simulink model "Engine_Start_harness"  (Simulink 7.7)
settings: Solver=FixedStepDiscrete  SolverMode=SingleTasking  StartTime=0.0  StopTime=100  FixedStep=0.01  RelTol=1e-3
PostLoadFcn:
  | load EngineStart.mat
undefined symbols (not defined in the file): ACTIVE, INACTIVE, NORMAL, SA_ATTACHMENT, SA_SERVICE_TOOL, sigbuilder_block, srate
CloseFcn:
  | rtwprivate ssgencode ModelCloseRequest sle_main_controller
settings Model: Creator=smindema  LastModifiedBy=aliebel  RecordCoverage=on  CovMetricSettings=dcmw  CovCumulativeReport=on  CovModelRefEnable=off
settings MATStruct: SampleTime=0.01  Offset=0  Priority=[1.0]
settings DataIOCC: LimitDataPoints=off  SaveOutput=off  SaveTime=off
settings OptimizationCC: BlockReduction=off  InlineParams=on  ExpressionFolding=off  StateBitsets=on  DataBitsets=on  UseTempVars=on  InitFltsAndDblsToZero=on  NoFixptDivByZeroProtection=on  EfficientFloat2IntCast=on  OptimizeModelRefInitCode=on
settings DebuggingCC: SaveWithParameterizedLinksMsg=none  MultiTaskDSMMsg=warning  MultiTaskCondExecSysMsg=none  IntegerOverflowMsg=none  ModelReferenceCSMismatchMessage=warning
settings HardwareCC: ProdBitPerInt=16  ProdBitPerPointer=16  ProdIntDivRoundTo=Floor  ProdEndianess=BigEndian  ProdWordSize=16  ProdHWDeviceType=Motorola HC12
settings ModelReferenceCC: ModelReferenceNumInstancesAllowed=Single
settings RTWCC: SystemTargetFile=ert.tlc  GenCodeOnly=on  TemplateMakefile=ert_default_tmf  Description=Real-Time Workshop Embedded Coder (no auto configuration)  GenerateReport=on  RetainRTWFile=on  ProcessScript=ert_make_rtw_hook  IncludeHyperlinkInReport=on  LaunchReport=on  IncludeERTFirstTime=on
settings RTWCC: CustomHeaderCode=|
  | #include "cpp_req_defines.h"
  | #include "hw_fin.h"
  | #include "cdata.h"
settings CodeAppCC: IgnoreCustomStorageClasses=off  DefineNamingRule=UpperCase
settings ERTTargetCC: TargetFcnLib=ansi_tfl_tmw.mat  FunctionExecutionProfile=off  MultiwordLength=2048  GenerateSampleERTMain=on  IncludeMdlTerminateFcn=off  SupportAbsoluteTime=off  SupportNonFinite=off  SupportComplex=off  PurelyIntegerCode=on  ERTCustomFileTemplate=gen_rtw_req_defines_h.tlc  GlobalDataDefinition=InSeparateSourceFile  GlobalDataReference=InSeparateHeaderFile  ConvertIfToSwitch=off

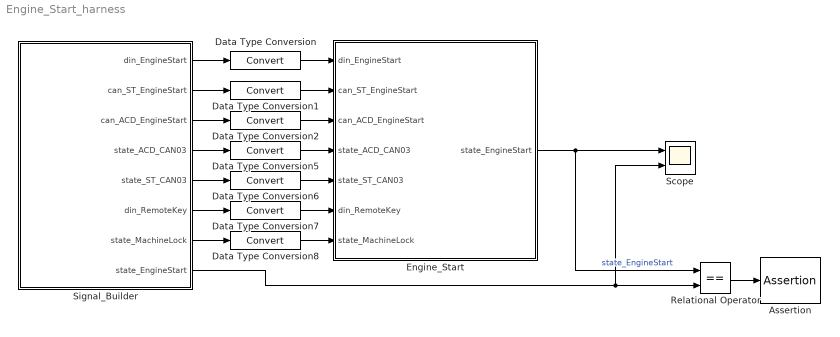
== system Engine_Start_harness ==
  Assertion : Assertion  Enabled=off
  Data Type Conversion{,1..2,5..8} (7 alike) : DataTypeConversion
  Engine_Start : Subsystem  TreatAsAtomicUnit=on  SystemSampleTime=srate  RTWFcnName=Engine_Start  RTWFileName=mod_Inputs
      settings: RTWSystemCode=Function  RTWFcnNameOpts=User specified  RTWFileNameOpts=User specified
  Relational Operator : RelationalOperator  Operator===  OutDataTypeStr=boolean
  Scope : Scope  NumInputPorts=2
      settings: YMin=-5~-5  YMax=5~5  MaxDataPoints=50000
  Signal_Builder : Subsystem  Tag=STV Subsys  LoadFcn=sigbuilder_block('load');  StartFcn=sigbuilder_block('start');  StopFcn=sigbuilder_block('stop');  ClipboardFcn=sigbuilder_block('clipboard');  mask(Sigbuilder block){}
      mask help: Sigbuilder GUI
      mask init:
      | if ~strcmp(get_param(bdroot(gcbh),'SimulationStatus'),'stopped') tuvar = sigbuilder_block('maskInit'); end
      settings: CopyFcn=sigbuilder_block('copy');  DeleteFcn=sigbuilder_block('delete');  ModelCloseFcn=sigbuilder_block('modelClose');  PreSaveFcn=sigbuilder_block('preSave');  NameChangeFcn=sigbuilder_block('namechange');  OpenFcn=sigbuilder_block('open',[91.5 225.75 1119.75 509.25 ]);  CloseFcn=sigbuilder_block('close');
      mask Display: plot(0,0,100,100,[10,10,40,40,10],[80,20,20,80,80],[40,10],[50,50], [40,27,10],[65,72,56],[40,25,25,10],[28,28,43,43]);
  wires:
  Engine_Start/1(state_EngineStart) -> Scope/1, Relational Operator/1  "state_EngineStart"
  Signal_Builder/1(din_EngineStart) -> Data Type Conversion/1
  Signal_Builder/2(can_ST_EngineStart) -> Data Type Conversion1/1
  Data Type Conversion/1 -> Engine_Start/1(din_EngineStart)
  Data Type Conversion1/1 -> Engine_Start/2(can_ST_EngineStart)
  Relational Operator/1 -> Assertion/1
  Data Type Conversion2/1 -> Engine_Start/3(can_ACD_EngineStart)
  Signal_Builder/3(can_ACD_EngineStart) -> Data Type Conversion2/1
  Signal_Builder/4(state_ACD_CAN03) -> Data Type Conversion5/1
  Signal_Builder/5(state_ST_CAN03) -> Data Type Conversion6/1
  Data Type Conversion5/1 -> Engine_Start/4(state_ACD_CAN03)
  Data Type Conversion6/1 -> Engine_Start/5(state_ST_CAN03)
  Signal_Builder/6(din_RemoteKey) -> Data Type Conversion7/1
  Signal_Builder/7(state_MachineLock) -> Data Type Conversion8/1
  Data Type Conversion7/1 -> Engine_Start/6(din_RemoteKey)
  Data Type Conversion8/1 -> Engine_Start/7(state_MachineLock)
  Signal_Builder/8(state_EngineStart) -> Relational Operator/2, Scope/2

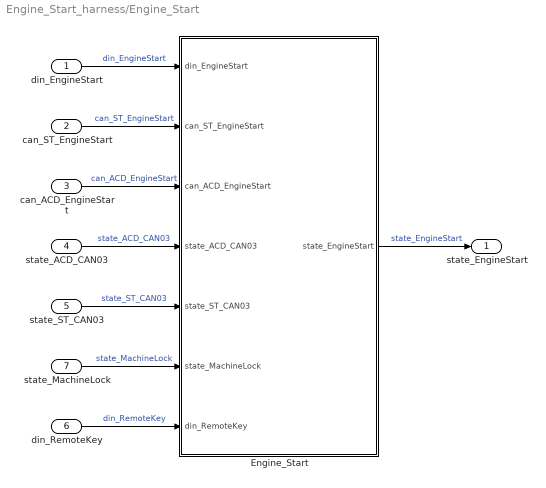
== system Engine_Start_harness/Engine_Start ==
  din_EngineStart : Inport
  can_ST_EngineStart : Inport  Port=2
  can_ACD_EngineStart : Inport  Port=3
  state_ACD_CAN03 : Inport  Port=4
  state_ST_CAN03 : Inport  Port=5
  din_RemoteKey : Inport  Port=6
  state_MachineLock : Inport  Port=7
  Engine_Start : Stateflow chart  TreatAsAtomicUnit=on
  state_EngineStart : Outport
  wires:
  Engine_Start/1(state_EngineStart) -> state_EngineStart/1  "state_EngineStart"
  din_EngineStart/1 -> Engine_Start/1(din_EngineStart)  "din_EngineStart"
  can_ST_EngineStart/1 -> Engine_Start/2(can_ST_EngineStart)  "can_ST_EngineStart"
  can_ACD_EngineStart/1 -> Engine_Start/3(can_ACD_EngineStart)  "can_ACD_EngineStart"
  state_ACD_CAN03/1 -> Engine_Start/4(state_ACD_CAN03)  "state_ACD_CAN03"
  state_ST_CAN03/1 -> Engine_Start/5(state_ST_CAN03)  "state_ST_CAN03"
  state_MachineLock/1 -> Engine_Start/6(state_MachineLock)  "state_MachineLock"
  din_RemoteKey/1 -> Engine_Start/7(din_RemoteKey)  "din_RemoteKey"

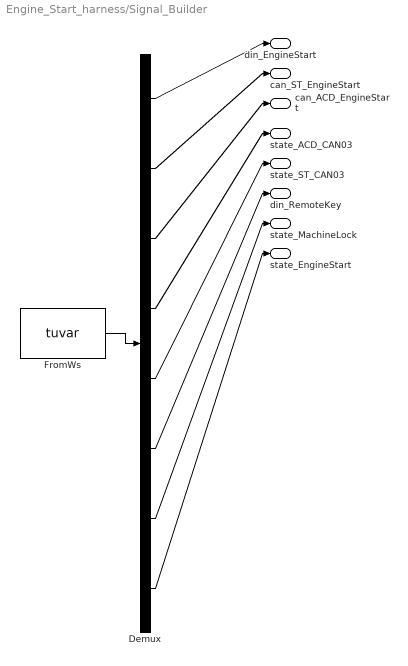
== system Engine_Start_harness/Signal_Builder ==
  Demux : Demux  Tag=STV Demux  Outputs=8
  FromWs : FromWorkspace  Tag=STV FromWs  VariableName=tuvar  SampleTime=0  SigBuilderData=DataTag0  VnvData=DataTag1
      SigBuilderData=|
      | common.afterFinalStr = 'Extrapolate'
      | common.sampleTime = 0
      | dataSet.timeRange = [0 100]
      | dataSet.name = 'T1-Key'
      | sbobj.Groups.Name = 'T1-Key'
      | sbobj.Groups.Signals(1).Name = 'din_EngineStart'
      | sbobj.Groups.Signals(1).XData = [0 4.8 4.8 8.3 8.3 13.9 13.9 17.8 17.8 23.7 23.7 28 28 100]
      | sbobj.Groups.Signals(1).YData = [0 0 1 1 0 0 1 1 0 0 1 1 0 0]
      | sbobj.Groups.Signals(2).Name = 'can_ST_EngineStart'
      | sbobj.Groups.Signals(2).XData = [0 30 30 35 35 40 40 45 45 100]
      | sbobj.Groups.Signals(2).YData = [0 0 1 1 0 0 1 1 0 0]
      | sbobj.Groups.Signals(3).Name = 'can_ACD_EngineStart'
      | sbobj.Groups.Signals(3).XData = [0 50 50 54.5 54.5 60 60 65 65 100]
      | sbobj.Groups.Signals(3).YData = [0 0 1 1 0 0 1 1 0 0]
      | sbobj.Groups.Signals(4).Name = 'state_ACD_CAN03'
      | sbobj.Groups.Signals(4).XData = [0 52 52 62.7 62.7 100]
      | sbobj.Groups.Signals(4).YData = [4 4 8 8 4 4]
      | sbobj.Groups.Signals(5).Name = 'state_ST_CAN03'
      | sbobj.Groups.Signals(5).XData = [0 32.8 32.8 42 42 100]
      | sbobj.Groups.Signals(5).YData = [4 4 8 8 4 4]
      | sbobj.Groups.Signals(6).Name = 'din_RemoteKey'
      | sbobj.Groups.Signals(6).XData = [0 11.1 11.1 19.8 19.8 100]
      | sbobj.Groups.Signals(6).YData = [0 0 1 1 0 0]
      | sbobj.Groups.Signals(7).Name = 'state_MachineLock'
      | sbobj.Groups.Signals(7).XData = [0 10 10 100]
      | sbobj.Groups.Signals(7).YData = [1 1 0 0]
      | sbobj.Groups.Signals(8).Name = 'state_EngineStart'
      | sbobj.Groups.Signals(8).XData = [0 23.71 23.71 28 28 32.81 32.81 35 35 40 40 42 42 52 52 54.5 54.5 60 60 62.7 62.7 100]
      | sbobj.Groups.Signals(8).YData = [0 0 1 1 0 0 1 1 0 0 1 1 0 0 1 1 0 0 1 1 0 0]
  din_EngineStart : Outport  Tag=STV Outport
  can_ST_EngineStart : Outport  Tag=STV Outport  Port=2
  can_ACD_EngineStart : Outport  Tag=STV Outport  Port=3
  state_ACD_CAN03 : Outport  Tag=STV Outport  Port=4
  state_ST_CAN03 : Outport  Tag=STV Outport  Port=5
  din_RemoteKey : Outport  Tag=STV Outport  Port=6
  state_MachineLock : Outport  Tag=STV Outport  Port=7
  state_EngineStart : Outport  Tag=STV Outport  Port=8
  wires:
  FromWs/1 -> Demux/1
  Demux/1 -> din_EngineStart/1
  Demux/2 -> can_ST_EngineStart/1
  Demux/3 -> can_ACD_EngineStart/1
  Demux/4 -> state_ACD_CAN03/1
  Demux/5 -> state_ST_CAN03/1
  Demux/6 -> din_RemoteKey/1
  Demux/7 -> state_MachineLock/1
  Demux/8 -> state_EngineStart/1

== stateflow chart Engine_Start/Engine_Start ==
  state OFF
    en:state_EngineStart = INACTIVE;
  state ON
    en:state_EngineStart = ACTIVE;
  (default) -> OFF
  OFF -> (junction 5)
  (junction 6) -> OFF [order 3] : [(start_Device == SA_ATTACHMENT)...
      | && ((can_ACD_EngineStart != ACTIVE) || (state_ACD_CAN03 != NORMAL))]
  (junction 5) -> ON [order 2] : [(can_ST_EngineStart == ACTIVE)...
      | && (state_ST_CAN03 == NORMAL)]
      | {
      | start_Device = SA_SERVICE_TOOL;
      | }
  (junction 5) -> ON [order 3] : [(can_ACD_EngineStart == ACTIVE)...
      | && (state_ACD_CAN03 == NORMAL)]
      | {
      | start_Device = SA_ATTACHMENT;
      | }
  (junction 6) -> OFF [order 1] : [(start_Device == SA_SERVICE_TOOL)...
      | && ((can_ST_EngineStart != ACTIVE) || (state_ST_CAN03 != NORMAL))]
  ON -> (junction 6)
  (junction 6) -> OFF [order 2] : [(start_Device == 0)...
      | && (din_EngineStart == INACTIVE)]
  (junction 5) -> ON [order 1] : [(din_EngineStart == ACTIVE)...
      | && (state_MachineLock != ACTIVE)...
      | && (din_RemoteKey != ACTIVE)]
      | {
      | start_Device = 0;
      | }
  data: din_EngineStart input uint8; can_ST_EngineStart input uint8; state_EngineStart output uint8 =0; INACTIVE parameter uint8 =0; ACTIVE parameter uint8 =1; can_ACD_EngineStart input uint8; state_ACD_CAN03 input uint8; state_ST_CAN03 input uint8; SA_SERVICE_TOOL parameter uint8; SA_ATTACHMENT parameter uint8; start_Device local uint8; NORMAL parameter uint8 =1; state_MachineLock input uint8; din_RemoteKey input uint8
